simulink model "AutoDRIVE_RZR_AEB"  (R2024b)
settings: Solver=FixedStepAuto  StartTime=0.0  StopTime=180  RelTol=1e-3
settings Model: DataDictionary=DataDictionary.sldd  VariantConfigurationObject=Variants  Creator=csamak  LastModifiedBy=tsamak
settings OptimizationCC: ZeroExternalMemoryAtStartup=off  ZeroInternalMemoryAtStartup=off  InitFltsAndDblsToZero=on
settings DebuggingCC: AlgebraicLoopMsg=none
settings HardwareCC: ProdLongLongMode=on  TargetLongLongMode=on
settings RTWCC: TargetLang=C++  GenerateGPUCode=CUDA
settings GRTTargetCC: TargetLangStandard=C++11 (ISO)  CodeInterfacePackaging=C++ class

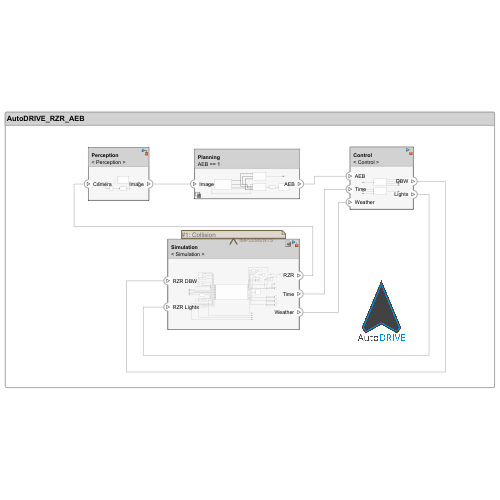
[thumbnail: Simulink's stored preview of the top-level diagram]
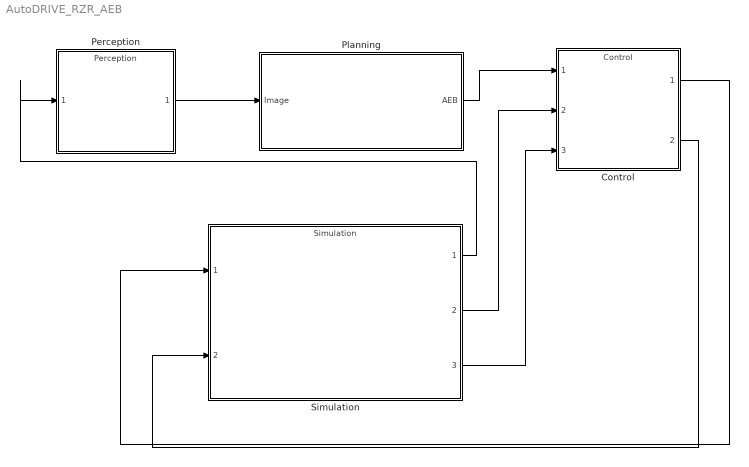
== system AutoDRIVE_RZR_AEB ==
  Control : ModelReference  ModelNameDialog=Control  SimulationMode=Normal  ModelReferenceVersion=1.14
      settings: PortSchema="{\"entries\":[{\"content\":{\"headerSize\":38,\"margin\":15,\"minimumSpacing\":25,\"sides\":[{\"content\":{\"connectorIds\":[\"In1\",\"In2\",\"In3\"]},\"type\":\"ConnectorPlacement.EquallySpacedRectSide\",\"uuid\":\"28628df5-70f8-4fca-a249-e40856b928d2\"},{\"content\":{\"connectorIds\":[\"Out1\",\"Out2\"],\"side\":\"RIGHT\"},\"type\":\"ConnectorPlacement.EquallySpacedRectSide\",\"uuid\":\"bb51d37c-ccb1-462c-be18-3bafe046c964\"},{\"content\":{\"side\":\"TOP\"},\"type\":\"ConnectorPlacement.EquallySpacedRectSide\",\"uuid\":\"7ff12ae2-9fd6-4f30-a5f3-c2b2b7907720\"}]},\"type\":\"ConnectorPlacement.EquallySpacedConnector\",\"uuid\":\"e5210a3c-b91d-4543-8d12-66c28dc06f32\"}],\"packageUris\":[\"http://schema.mathworks.com/mf0/Connector/R2020b\"],\"version\":\"1.0\"}"
  Perception : ModelReference  ModelNameDialog=Perception  SimulationMode=Normal  ModelReferenceVersion=1.9
      settings: PortSchema="{\"entries\":[{\"content\":{\"headerSize\":38,\"margin\":15,\"minimumSpacing\":25,\"sides\":[{\"content\":{\"connectorIds\":[\"In1\"]},\"type\":\"ConnectorPlacement.EquallySpacedRectSide\",\"uuid\":\"28628df5-70f8-4fca-a249-e40856b928d2\"},{\"content\":{\"connectorIds\":[\"Out1\"],\"side\":\"RIGHT\"},\"type\":\"ConnectorPlacement.EquallySpacedRectSide\",\"uuid\":\"bb51d37c-ccb1-462c-be18-3bafe046c964\"},{\"content\":{\"side\":\"TOP\"},\"type\":\"ConnectorPlacement.EquallySpacedRectSide\",\"uuid\":\"7ff12ae2-9fd6-4f30-a5f3-c2b2b7907720\"}]},\"type\":\"ConnectorPlacement.EquallySpacedConnector\",\"uuid\":\"e5210a3c-b91d-4543-8d12-66c28dc06f32\"}],\"packageUris\":[\"http://schema.mathworks.com/mf0/Connector/R2020b\"],\"version\":\"1.0\"}"
  Planning : Subsystem  Variant=on  VariantControlMode=label  LabelModeActiveChoice=AEB == 1
      settings: PortSchema="{\"entries\":[{\"content\":{\"headerSize\":38,\"margin\":15,\"minimumSpacing\":25,\"sides\":[{\"content\":{\"connectorIds\":[\"In1\"]},\"type\":\"ConnectorPlacement.EquallySpacedRectSide\",\"uuid\":\"f44ffee4-899a-4ca9-ac35-010cf54653fa\"},{\"content\":{\"connectorIds\":[\"Out1\"],\"side\":\"RIGHT\"},\"type\":\"ConnectorPlacement.EquallySpacedRectSide\",\"uuid\":\"e40c10fd-dcc2-4178-ab03-520b5ac0ff55\"},{\"content\":{\"side\":\"TOP\"},\"type\":\"ConnectorPlacement.EquallySpacedRectSide\",\"uuid\":\"96049f6c-5e58-4217-9fe6-d37131842aed\"}]},\"type\":\"ConnectorPlacement.EquallySpacedConnector\",\"uuid\":\"0fb3cb18-c4d3-4902-8ca1-5c2ccd8c790c\"}],\"packageUris\":[\"http://schema.mathworks.com/mf0/Connector/R2020b\"],\"version\":\"1.0\"}"
  Simulation : ModelReference  ModelNameDialog=Simulation  SimulationMode=Normal  ModelReferenceVersion=1.25
      settings: PortSchema="{\"entries\":[{\"content\":{\"headerSize\":38,\"margin\":15,\"minimumSpacing\":25,\"sides\":[{\"content\":{\"connectorIds\":[\"In1\",\"In2\"]},\"type\":\"ConnectorPlacement.EquallySpacedRectSide\",\"uuid\":\"fafa5590-994c-41ae-98dd-b3fdf6cfc728\"},{\"content\":{\"connectorIds\":[\"Out1\",\"Out2\",\"Out3\"],\"side\":\"RIGHT\"},\"type\":\"ConnectorPlacement.EquallySpacedRectSide\",\"uuid\":\"9ced0dfe-3d4e-4aa4-8870-59bd0423e1a3\"},{\"content\":{\"side\":\"TOP\"},\"type\":\"ConnectorPlacement.EquallySpacedRectSide\",\"uuid\":\"b746270d-efc5-4d25-8271-0b70c8bdfd8f\"}]},\"type\":\"ConnectorPlacement.EquallySpacedConnector\",\"uuid\":\"68d888a7-0c4c-4b63-b659-5a4d61de606b\"}],\"packageUris\":[\"http://schema.mathworks.com/mf0/Connector/R2020b\"],\"version\":\"1.0\"}"
  wires:
  Planning/1(AEB) -> Control/1
  Control/1 -> Simulation/1
  Control/2 -> Simulation/2
  Simulation/1 -> Perception/1
  Simulation/2 -> Control/2
  Simulation/3 -> Control/3
  Perception/1 -> Planning/1(Image)

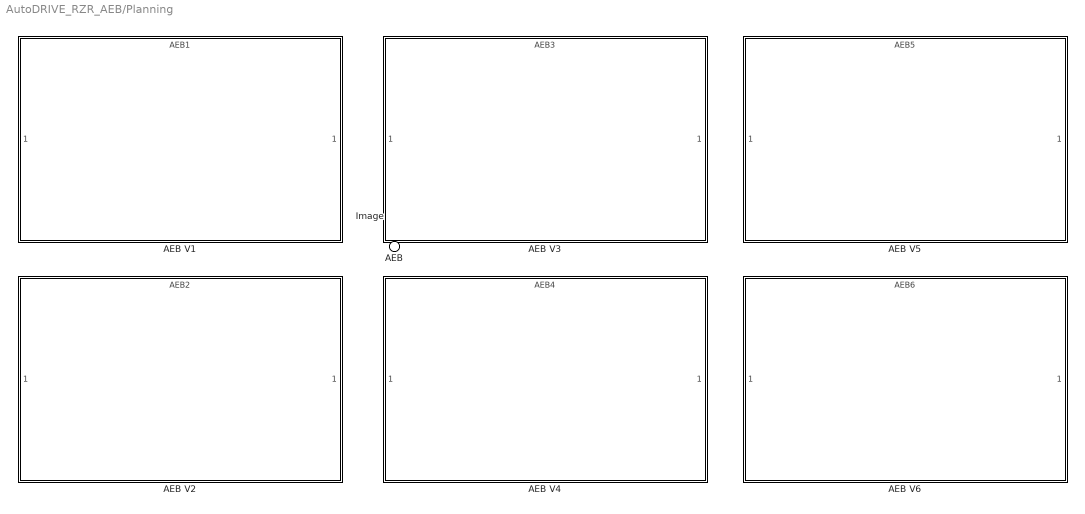
== system AutoDRIVE_RZR_AEB/Planning ==
  Image : Inport
  AEB V1 : ModelReference  ModelNameDialog=AEB1  SimulationMode=Normal  VariantControl=AEB == 1  ModelReferenceVersion=1.25
      settings: PortSchema="{\"entries\":[{\"content\":{\"headerSize\":38,\"margin\":15,\"minimumSpacing\":25,\"sides\":[{\"content\":{\"connectorIds\":[\"In1\"]},\"type\":\"ConnectorPlacement.EquallySpacedRectSide\",\"uuid\":\"28628df5-70f8-4fca-a249-e40856b928d2\"},{\"content\":{\"connectorIds\":[\"Out1\"],\"side\":\"RIGHT\"},\"type\":\"ConnectorPlacement.EquallySpacedRectSide\",\"uuid\":\"bb51d37c-ccb1-462c-be18-3bafe046c964\"},{\"content\":{\"side\":\"TOP\"},\"type\":\"ConnectorPlacement.EquallySpacedRectSide\",\"uuid\":\"7ff12ae2-9fd6-4f30-a5f3-c2b2b7907720\"}]},\"type\":\"ConnectorPlacement.EquallySpacedConnector\",\"uuid\":\"e5210a3c-b91d-4543-8d12-66c28dc06f32\"}],\"packageUris\":[\"http://schema.mathworks.com/mf0/Connector/R2020b\"],\"version\":\"1.0\"}"
  AEB V2 : ModelReference  ModelNameDialog=AEB2  SimulationMode=Normal  VariantControl=AEB == 2  ModelReferenceVersion=1.17
      settings: PortSchema="{\"entries\":[{\"content\":{\"headerSize\":38,\"margin\":15,\"minimumSpacing\":25,\"sides\":[{\"content\":{\"connectorIds\":[\"In1\"]},\"type\":\"ConnectorPlacement.EquallySpacedRectSide\",\"uuid\":\"28628df5-70f8-4fca-a249-e40856b928d2\"},{\"content\":{\"connectorIds\":[\"Out1\"],\"side\":\"RIGHT\"},\"type\":\"ConnectorPlacement.EquallySpacedRectSide\",\"uuid\":\"bb51d37c-ccb1-462c-be18-3bafe046c964\"},{\"content\":{\"side\":\"TOP\"},\"type\":\"ConnectorPlacement.EquallySpacedRectSide\",\"uuid\":\"7ff12ae2-9fd6-4f30-a5f3-c2b2b7907720\"}]},\"type\":\"ConnectorPlacement.EquallySpacedConnector\",\"uuid\":\"e5210a3c-b91d-4543-8d12-66c28dc06f32\"}],\"packageUris\":[\"http://schema.mathworks.com/mf0/Connector/R2020b\"],\"version\":\"1.0\"}"
  AEB V3 : ModelReference  ModelNameDialog=AEB3  SimulationMode=Normal  VariantControl=AEB == 3  ModelReferenceVersion=1.15
      settings: PortSchema="{\"entries\":[{\"content\":{\"headerSize\":38,\"margin\":15,\"minimumSpacing\":25,\"sides\":[{\"content\":{\"connectorIds\":[\"In1\"]},\"type\":\"ConnectorPlacement.EquallySpacedRectSide\",\"uuid\":\"28628df5-70f8-4fca-a249-e40856b928d2\"},{\"content\":{\"connectorIds\":[\"Out1\"],\"side\":\"RIGHT\"},\"type\":\"ConnectorPlacement.EquallySpacedRectSide\",\"uuid\":\"bb51d37c-ccb1-462c-be18-3bafe046c964\"},{\"content\":{\"side\":\"TOP\"},\"type\":\"ConnectorPlacement.EquallySpacedRectSide\",\"uuid\":\"7ff12ae2-9fd6-4f30-a5f3-c2b2b7907720\"}]},\"type\":\"ConnectorPlacement.EquallySpacedConnector\",\"uuid\":\"e5210a3c-b91d-4543-8d12-66c28dc06f32\"}],\"packageUris\":[\"http://schema.mathworks.com/mf0/Connector/R2020b\"],\"version\":\"1.0\"}"
  AEB V4 : ModelReference  ModelNameDialog=AEB4  SimulationMode=Normal  VariantControl=AEB == 4  ModelReferenceVersion=1.14
      settings: PortSchema="{\"entries\":[{\"content\":{\"headerSize\":38,\"margin\":15,\"minimumSpacing\":25,\"sides\":[{\"content\":{\"connectorIds\":[\"In1\"]},\"type\":\"ConnectorPlacement.EquallySpacedRectSide\",\"uuid\":\"28628df5-70f8-4fca-a249-e40856b928d2\"},{\"content\":{\"connectorIds\":[\"Out1\"],\"side\":\"RIGHT\"},\"type\":\"ConnectorPlacement.EquallySpacedRectSide\",\"uuid\":\"bb51d37c-ccb1-462c-be18-3bafe046c964\"},{\"content\":{\"side\":\"TOP\"},\"type\":\"ConnectorPlacement.EquallySpacedRectSide\",\"uuid\":\"7ff12ae2-9fd6-4f30-a5f3-c2b2b7907720\"}]},\"type\":\"ConnectorPlacement.EquallySpacedConnector\",\"uuid\":\"e5210a3c-b91d-4543-8d12-66c28dc06f32\"}],\"packageUris\":[\"http://schema.mathworks.com/mf0/Connector/R2020b\"],\"version\":\"1.0\"}"
  AEB V5 : ModelReference  ModelNameDialog=AEB5  SimulationMode=Normal  VariantControl=AEB == 5  ModelReferenceVersion=1.14
      settings: PortSchema="{\"entries\":[{\"content\":{\"headerSize\":38,\"margin\":15,\"minimumSpacing\":25,\"sides\":[{\"content\":{\"connectorIds\":[\"In1\"]},\"type\":\"ConnectorPlacement.EquallySpacedRectSide\",\"uuid\":\"28628df5-70f8-4fca-a249-e40856b928d2\"},{\"content\":{\"connectorIds\":[\"Out1\"],\"side\":\"RIGHT\"},\"type\":\"ConnectorPlacement.EquallySpacedRectSide\",\"uuid\":\"bb51d37c-ccb1-462c-be18-3bafe046c964\"},{\"content\":{\"side\":\"TOP\"},\"type\":\"ConnectorPlacement.EquallySpacedRectSide\",\"uuid\":\"7ff12ae2-9fd6-4f30-a5f3-c2b2b7907720\"}]},\"type\":\"ConnectorPlacement.EquallySpacedConnector\",\"uuid\":\"e5210a3c-b91d-4543-8d12-66c28dc06f32\"}],\"packageUris\":[\"http://schema.mathworks.com/mf0/Connector/R2020b\"],\"version\":\"1.0\"}"
  AEB V6 : ModelReference  ModelNameDialog=AEB6  SimulationMode=Normal  VariantControl=AEB == 6  ModelReferenceVersion=1.19
      settings: PortSchema="{\"entries\":[{\"content\":{\"headerSize\":38,\"margin\":15,\"minimumSpacing\":25,\"sides\":[{\"content\":{\"connectorIds\":[\"In1\"]},\"type\":\"ConnectorPlacement.EquallySpacedRectSide\",\"uuid\":\"28628df5-70f8-4fca-a249-e40856b928d2\"},{\"content\":{\"connectorIds\":[\"Out1\"],\"side\":\"RIGHT\"},\"type\":\"ConnectorPlacement.EquallySpacedRectSide\",\"uuid\":\"bb51d37c-ccb1-462c-be18-3bafe046c964\"},{\"content\":{\"side\":\"TOP\"},\"type\":\"ConnectorPlacement.EquallySpacedRectSide\",\"uuid\":\"7ff12ae2-9fd6-4f30-a5f3-c2b2b7907720\"}]},\"type\":\"ConnectorPlacement.EquallySpacedConnector\",\"uuid\":\"e5210a3c-b91d-4543-8d12-66c28dc06f32\"}],\"packageUris\":[\"http://schema.mathworks.com/mf0/Connector/R2020b\"],\"version\":\"1.0\"}"
  AEB : Outport
